simulink model "quadrotor_system"  (R2017a)
settings: Solver=ode1  StartTime=0.0  StopTime=10.0  FixedStep=0.001  RelTol=1e-3  EnableMultiTasking=on
values from neighbouring files (symbols this model uses):
  b = 3.13*10^(-5)    (= 3.13e-05)    [Quadparameters.m]    (also in Quadparameters2.m)
  d = 7.5*10^(-7)    (= 7.5e-07)    [Quadparameters.m]    (also in Quadparameters2.m)
  g = 9.807    [Quadparameters.m]    (also in Quadparameters2.m = 9.81)
  Ix = 7.5*10^(-3)    (= 0.0075)    [Quadparameters.m]    (also in Quadparameters2.m)
  Iy = 7.5*10^(-3)    (= 0.0075)    [Quadparameters.m]    (also in Quadparameters2.m)
  Iz = 1.3*10^(-2)    (= 0.013)    [Quadparameters.m]    (also in Quadparameters2.m)
  Jr = 6.5*10^(-5)    (= 6.5e-05)    [Quadparameters.m]    (also in Quadparameters2.m)
  l = 0.23    [Quadparameters.m]    (also in Quadparameters2.m)
  m = 0.65    [Quadparameters.m]    (also in Quadparameters2.m)
settings Model: Creator=j.wan  LastModifiedBy=jean-marie
settings DataIOCC: LimitDataPoints=on  SaveFormat=Array
settings DebuggingCC: SFUnexpectedBacktrackingDiag=warning  SFNoUnconditionalDefaultTransitionDiag=warning  SFExecutionAtInitializationDiag=none
settings HardwareCC: ProdBitPerPointer=32  ProdBitPerSizeT=32  ProdBitPerPtrDiffT=32  ProdLargestAtomicFloat=None  ProdIntDivRoundTo=Undefined  ProdEndianess=Unspecified  ProdWordSize=32  ProdHWDeviceType=32-bit Generic
settings ModelReferenceCC: PropagateSignalLabelsOutOfModel=off
settings RTWCC: SystemTargetFile=fmu_cs2.tlc  MakeCommand=make_rtw FMIT_INTERMEDIATE_LIB_DIR=DEFAULT FMIT_ADDITIONAL_CFLAGS=  TemplateMakefile=fmu_cs2_default_tmf  Description=FMU Co-Simulation 2.0 Standalone
settings STFCustomTargetCC: ModelReferenceCompliant=off  MATLABClassNameForMDSCustomization=Simulink.SoftwareTarget.TargetSpecificTriggerConfigurationBase  SystemTargetFile=fmu_cs2.tlc
settings ConfigComp: CovMetricSettings=dw  CovHtmlReporting=on  CovSaveCumulativeToWorkspaceVar=on  CovSaveSingleToWorkspaceVar=on  CovExternalEMLEnable=off

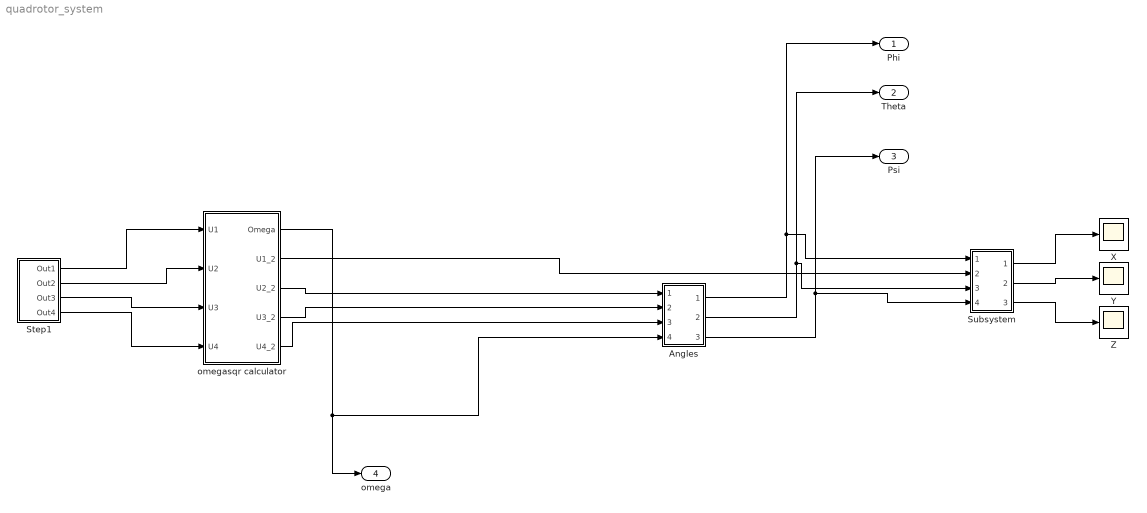
== system quadrotor_system ==
  Angles : Subsystem
  Step1 : Subsystem
  Subsystem : Subsystem
  X : Scope
  Y : Scope
  Z : Scope
  omegasqr calculator : Subsystem
  Phi : Outport
  Theta : Outport  Port=2
  Psi : Outport  Port=3
  omega : Outport  Port=4
  wires:
  omegasqr calculator/1(Omega) -> Angles/4(In4), omega/1
  Step1/1(Out1) -> omegasqr calculator/1(U1)
  Step1/2(Out2) -> omegasqr calculator/2(U2)
  Step1/3(Out3) -> omegasqr calculator/3(U3)
  Step1/4(Out4) -> omegasqr calculator/4(U4)
  Angles/2(Out2) -> Subsystem/3(In3), Theta/1
  Angles/1(Out1) -> Subsystem/1(In1), Phi/1
  Angles/3(Out3) -> Subsystem/4(In4), Psi/1
  omegasqr calculator/3(U2_2) -> Angles/1(In1)
  omegasqr calculator/4(U3_2) -> Angles/2(In2)
  omegasqr calculator/5(U4_2) -> Angles/3(In3)
  omegasqr calculator/2(U1_2) -> Subsystem/2(In2)
  Subsystem/1(Out1) -> X/1
  Subsystem/2(Out2) -> Y/1
  Subsystem/3(Out3) -> Z/1

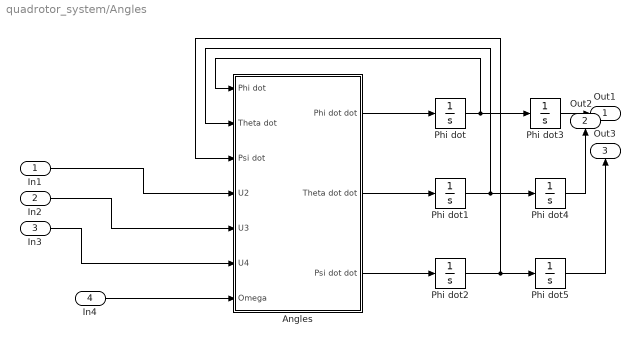
== system quadrotor_system/Angles ==
  In1 : Inport
  In2 : Inport  Port=2
  In3 : Inport  Port=3
  In4 : Inport  Port=4
  Angles : Subsystem
  Phi dot : Integrator
  Phi dot{1..5} (5 alike) : Integrator  ZeroCross=off
  Out1 : Outport
  Out2 : Outport  Port=2
  Out3 : Outport  Port=3
  wires:
  In4/1 -> Angles/7(Omega)
  Phi dot5/1 -> Out3/1
  Phi dot3/1 -> Out1/1
  Phi dot4/1 -> Out2/1
  In3/1 -> Angles/6(U4)
  Phi dot1/1 -> Angles/2(Theta dot), Phi dot4/1
  Phi dot2/1 -> Angles/3(Psi dot), Phi dot5/1
  In2/1 -> Angles/5(U3)
  In1/1 -> Angles/4(U2)
  Phi dot/1 -> Angles/1(Phi dot), Phi dot3/1
  Angles/1(Phi dot dot) -> Phi dot/1
  Angles/2(Theta dot dot) -> Phi dot1/1
  Angles/3(Psi dot dot) -> Phi dot2/1

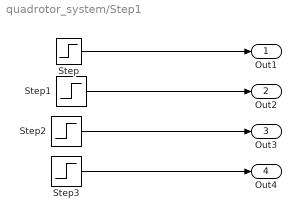
== system quadrotor_system/Step1 ==
  Step{,1..3} (4 alike) : Step  SampleTime=0
  Out1 : Outport
  Out2 : Outport  Port=2
  Out3 : Outport  Port=3
  Out4 : Outport  Port=4
  wires:
  Step2/1 -> Out3/1
  Step/1 -> Out1/1
  Step1/1 -> Out2/1
  Step3/1 -> Out4/1

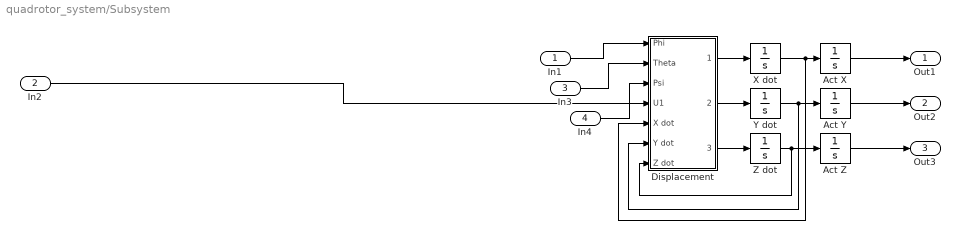
== system quadrotor_system/Subsystem ==
  In1 : Inport
  In2 : Inport  Port=2
  In3 : Inport  Port=3
  In4 : Inport  Port=4
  Act X : Integrator
  Act Y : Integrator
  Act Z : Integrator
  Displacement : Subsystem
  X dot : Integrator
  Y dot : Integrator
  Z dot : Integrator
  Out1 : Outport
  Out2 : Outport  Port=2
  Out3 : Outport  Port=3
  wires:
  Act Y/1 -> Out2/1
  Act Z/1 -> Out3/1
  Act X/1 -> Out1/1
  Y dot/1 -> Displacement/6(Y dot), Act Y/1
  X dot/1 -> Displacement/5(X dot), Act X/1
  Displacement/3(z dotdot) -> Z dot/1
  Z dot/1 -> Displacement/7(Z dot), Act Z/1
  Displacement/2(y dotdot) -> Y dot/1
  Displacement/1(x dotdot) -> X dot/1
  In2/1 -> Displacement/4(U1)
  In1/1 -> Displacement/1(Phi)
  In4/1 -> Displacement/3(Psi)
  In3/1 -> Displacement/2(Theta)

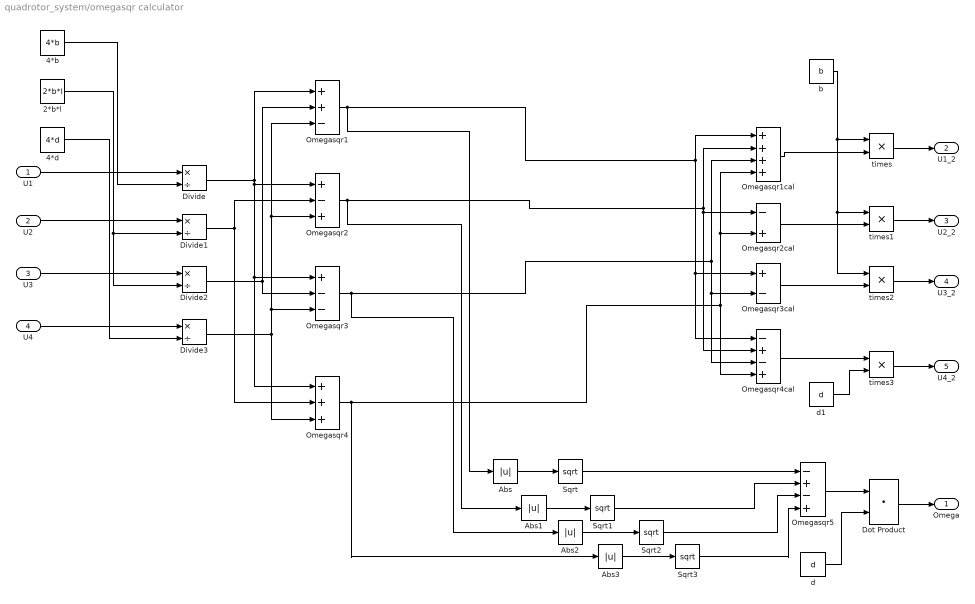
== system quadrotor_system/omegasqr calculator ==
  U1 : Inport
  U2 : Inport  Port=2
  U3 : Inport  Port=3
  U4 : Inport  Port=4
  2*b*l : Constant  Value=2*b*l
  4*b : Constant  Value=4*b
  4*d : Constant  Value=4*d
  Abs{,1..3} (4 alike) : Abs
  Divide{,1..3} (4 alike) : Product  Inputs=*/
  Dot Product : DotProduct  InputSameDT=on  OutDataTypeStr=Inherit: Inherit via internal rule
  Omegasqr1 : Sum  Inputs=++-
  Omegasqr1cal : Sum  Inputs=++++
  Omegasqr2 : Sum  Inputs=+-+
  Omegasqr2cal : Sum  Inputs=-+
  Omegasqr3 : Sum  Inputs=+--
  Omegasqr3cal : Sum  Inputs=+-
  Omegasqr4 : Sum  Inputs=+++
  Omegasqr4cal : Sum  Inputs=-+-+
  Omegasqr5 : Sum  Inputs=-+-+
  Sqrt{,1..3} (4 alike) : Sqrt  OutMin=[125]  OutMax=[523]  SaturateOnIntegerOverflow=on
  b : Constant  Value=b
  d : Constant  Value=d
  d1 : Constant  Value=d
  times{,1..3} (4 alike) : Product  Inputs=**
  Omega : Outport
  U1_2 : Outport  Port=2
  U2_2 : Outport  Port=3
  U3_2 : Outport  Port=4
  U4_2 : Outport  Port=5
  wires:
  U1/1 -> Divide/1
  4*b/1 -> Divide/2
  U2/1 -> Divide1/1
  2*b*l/1 -> Divide1/2, Divide2/2
  U3/1 -> Divide2/1
  U4/1 -> Divide3/1
  4*d/1 -> Divide3/2
  Divide/1 -> Omegasqr1/1, Omegasqr2/1, Omegasqr3/1, Omegasqr4/1
  Divide2/1 -> Omegasqr1/2, Omegasqr3/2
  Divide3/1 -> Omegasqr1/3, Omegasqr2/3, Omegasqr3/3, Omegasqr4/3
  Divide1/1 -> Omegasqr2/2, Omegasqr4/2
  Omegasqr1/1 -> Abs/1, Omegasqr1cal/1, Omegasqr3cal/1, Omegasqr4cal/1
  Omegasqr2/1 -> Abs1/1, Omegasqr1cal/2, Omegasqr2cal/1, Omegasqr4cal/2
  Omegasqr3/1 -> Abs2/1, Omegasqr1cal/3, Omegasqr3cal/2, Omegasqr4cal/3
  Omegasqr4/1 -> Abs3/1, Omegasqr1cal/4, Omegasqr2cal/2, Omegasqr4cal/4
  Omegasqr5/1 -> Dot Product/1
  Dot Product/1 -> Omega/1
  d/1 -> Dot Product/2
  b/1 -> times/1, times1/1, times2/1
  Omegasqr1cal/1 -> times/2
  Omegasqr2cal/1 -> times1/2
  Omegasqr3cal/1 -> times2/2
  Omegasqr4cal/1 -> times3/1
  d1/1 -> times3/2
  times/1 -> U1_2/1
  times1/1 -> U2_2/1
  times3/1 -> U4_2/1
  times2/1 -> U3_2/1
  Abs/1 -> Sqrt/1
  Abs1/1 -> Sqrt1/1
  Abs3/1 -> Sqrt3/1
  Abs2/1 -> Sqrt2/1
  Sqrt/1 -> Omegasqr5/1
  Sqrt1/1 -> Omegasqr5/2
  Sqrt2/1 -> Omegasqr5/3
  Sqrt3/1 -> Omegasqr5/4

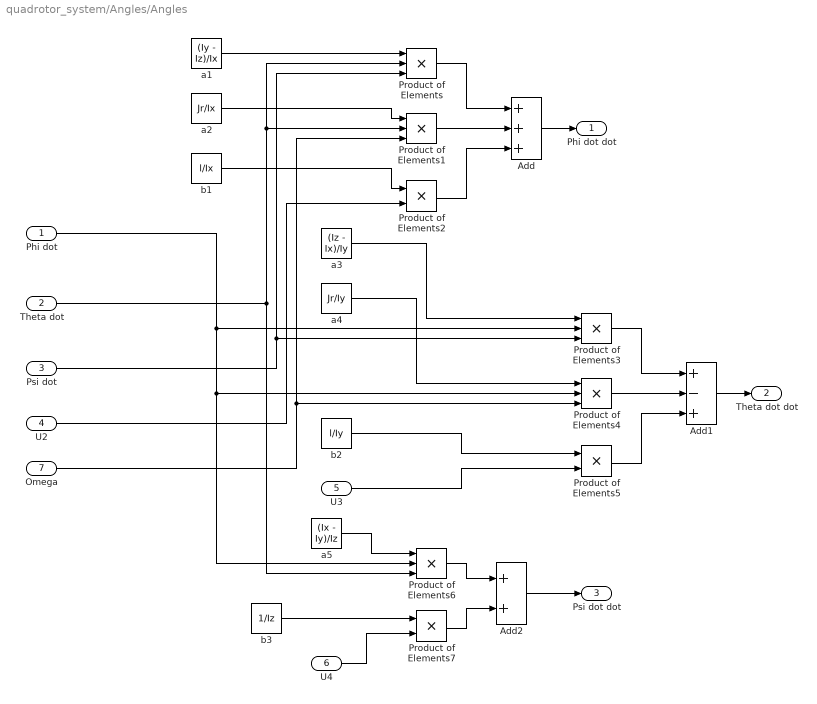
== system quadrotor_system/Angles/Angles ==
  Phi dot : Inport
  Theta dot : Inport  Port=2
  Psi dot : Inport  Port=3
  U2 : Inport  Port=4
  U3 : Inport  Port=5
  U4 : Inport  Port=6
  Omega : Inport  Port=7
  Add : Sum  Inputs=+++
  Add1 : Sum  Inputs=+-+
  Add2 : Sum
  Product of Elements{,1,3..4,6} (5 alike) : Product  Inputs=3
  Product of Elements2 : Product
  Product of Elements5 : Product
  Product of Elements7 : Product
  a1 : Constant  Value=(Iy - Iz)/Ix
  a2 : Constant  Value=Jr/Ix
  a3 : Constant  Value=(Iz - Ix)/Iy
  a4 : Constant  Value=Jr/Iy
  a5 : Constant  Value=(Ix - Iy)/Iz
  b1 : Constant  Value=l/Ix
  b2 : Constant  Value=l/Iy
  b3 : Constant  Value=1/Iz
  Phi dot dot : Outport
  Theta dot dot : Outport  Port=2
  Psi dot dot : Outport  Port=3
  wires:
  Product of Elements/1 -> Add/1
  Product of Elements1/1 -> Add/2
  Product of Elements2/1 -> Add/3
  Add/1 -> Phi dot dot/1
  a1/1 -> Product of Elements/1
  Theta dot/1 -> Product of Elements/2, Product of Elements1/2, Product of Elements6/3
  Psi dot/1 -> Product of Elements/3, Product of Elements3/3
  a2/1 -> Product of Elements1/1
  b1/1 -> Product of Elements2/1
  U2/1 -> Product of Elements2/2
  Omega/1 -> Product of Elements1/3, Product of Elements4/3
  Product of Elements3/1 -> Add1/1
  Product of Elements4/1 -> Add1/2
  Product of Elements5/1 -> Add1/3
  Add1/1 -> Theta dot dot/1
  a3/1 -> Product of Elements3/1
  a4/1 -> Product of Elements4/1
  b2/1 -> Product of Elements5/1
  U3/1 -> Product of Elements5/2
  Phi dot/1 -> Product of Elements3/2, Product of Elements4/2, Product of Elements6/2
  Product of Elements6/1 -> Add2/1
  Product of Elements7/1 -> Add2/2
  Add2/1 -> Psi dot dot/1
  U4/1 -> Product of Elements7/2
  b3/1 -> Product of Elements7/1
  a5/1 -> Product of Elements6/1

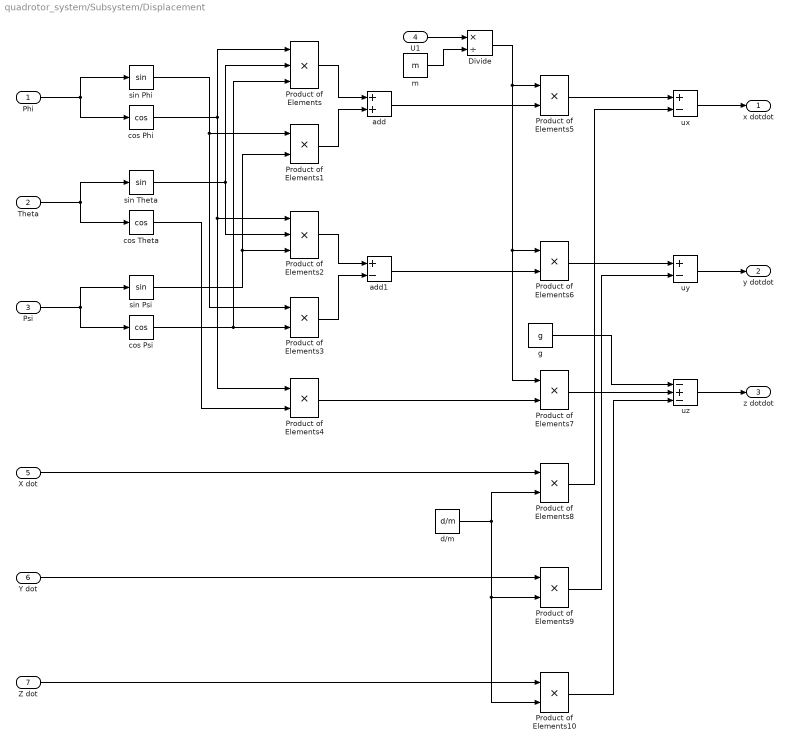
== system quadrotor_system/Subsystem/Displacement ==
  Phi : Inport
  Theta : Inport  Port=2
  Psi : Inport  Port=3
  U1 : Inport  Port=4
  X dot : Inport  Port=5
  Y dot : Inport  Port=6
  Z dot : Inport  Port=7
  Divide : Product  Inputs=*/
  Product of Elements : Product  Inputs=3
  Product of Elements{1,3..10} (9 alike) : Product
  Product of Elements2 : Product  Inputs=3
  add : Sum
  "add1 " : Sum  Inputs=+-
  cos Phi : Trigonometry  Operator=cos
  cos Psi : Trigonometry  Operator=cos
  cos Theta : Trigonometry  Operator=cos
  d/m : Constant  Value=d/m
  g : Constant  Value=g
  m : Constant  Value=m
  sin Phi : Trigonometry
  sin Psi : Trigonometry
  sin Theta : Trigonometry
  ux : Sum  Inputs=+-
  uy : Sum  Inputs=+-
  uz : Sum  Inputs=-+-
  x dotdot : Outport
  y dotdot : Outport  Port=2
  z dotdot : Outport  Port=3
  wires:
  Phi/1 -> sin Phi/1, cos Phi/1
  Theta/1 -> sin Theta/1, cos Theta/1
  Psi/1 -> sin Psi/1, cos Psi/1
  sin Theta/1 -> Product of Elements/2, Product of Elements2/2
  cos Psi/1 -> Product of Elements/3, Product of Elements3/2
  cos Phi/1 -> Product of Elements/1, Product of Elements2/1, Product of Elements4/1
  sin Phi/1 -> Product of Elements1/1, Product of Elements3/1
  sin Psi/1 -> Product of Elements1/2, Product of Elements2/3
  Product of Elements/1 -> add/1
  Product of Elements1/1 -> add/2
  add/1 -> Product of Elements5/2
  Product of Elements2/1 -> "add1 "/1
  Product of Elements3/1 -> "add1 "/2
  "add1 "/1 -> Product of Elements6/2
  cos Theta/1 -> Product of Elements4/2
  Product of Elements4/1 -> Product of Elements7/2
  U1/1 -> Divide/1
  m/1 -> Divide/2
  Divide/1 -> Product of Elements5/1, Product of Elements6/1, Product of Elements7/1
  Product of Elements5/1 -> ux/1
  Product of Elements6/1 -> uy/1
  uz/1 -> z dotdot/1
  Product of Elements7/1 -> uz/2
  g/1 -> uz/1
  X dot/1 -> Product of Elements8/1
  Y dot/1 -> Product of Elements9/1
  Z dot/1 -> Product of Elements10/1
  d/m/1 -> Product of Elements8/2, Product of Elements10/2, Product of Elements9/2
  Product of Elements10/1 -> uz/3
  Product of Elements8/1 -> ux/2
  Product of Elements9/1 -> uy/2
  ux/1 -> x dotdot/1
  uy/1 -> y dotdot/1
